simulink model "deneme"  (R2021a)
settings: Solver=FixedStepDiscrete  StartTime=0.0  StopTime=2  RelTol=1e-3  EnableMultiTasking=on
InitFcn:
  | pull_data ;
model workspace (MAT data in the model file):
  encoderResolution = 2000
  hallOffset = '0.5'
  indexOffset = 850
  polePairs = '4'
values from neighbouring files (symbols this model uses):
  bldc = mcb_bldc_param    [pull_data.m]
  dataType = 'single'    [pull_data.m]
  inverter = mcb_updateInverterParameters(bldc,inverter,target)    [pull_data.m]
  PI_params = mcb.internal.SetControllerParameters(bldc,inverter,PU_System,T_pwm,2*Ts,Ts_speed)    [pull_data.m]
  PU_System = mcb_SetPUSystem(bldc,inverter)    [pull_data.m]
  PWM_frequency = 20e3    (= 20000)    [pull_data.m]
  target = mcb_SetProcessorDetails('F28379D',PWM_frequency)    [pull_data.m]
  Ts = T_pwm    (= 5e-05)    [pull_data.m]
  Ts_motor = T_pwm/2    (= 2.5e-05)    [pull_data.m]
  Ts_motor_simscape = T_pwm/100    (= 5e-07)    [pull_data.m]
  Ts_simulink = T_pwm/2    (= 2.5e-05)    [pull_data.m]
  Ts_speed = 10*Ts    (= 0.0005)    [pull_data.m]
undefined symbols (not defined in the file or in its folder): Down, GPTRIP1SEL, GPTRIP2SEL, TZ1, TZ2, Up
libraries: nesl_utility x15, simulink x14, fl_lib x10, c2802xlib x9, mcbcontrolslib x8, c280xlib x6, mcbpositiondecoderlib x5, c2837xDlib x5, ee_lib x5, c2000lib x1, svdutilitieslib x1
(part 2 of 3)

== system deneme/Current Control/SCI (Code Generation)/Data_Logging ==
  note: Fast Serial Data Monitoring (32-bit)
  Data_Log : Inport
  Counter Limited : simulink/Sources/Counter Limited  uplimit=600-1  tsamp=-1
  Data : Subsystem  TreatAsAtomicUnit=on
  End : Subsystem  TreatAsAtomicUnit=on
  If : If  IfExpression=u1 == 0  ElseIfExpressions=u1 == 599
  Merge : Merge  Inputs=3
  Merge1 : Merge  Inputs=3
  Mux : Mux  Inputs=2
  Start : Subsystem  TreatAsAtomicUnit=on
  Width : Width  OutDataTypeMode=All ports same datatype  DataType=uint16
  SCI_Tx : Outport
  wires:
  If/3 -> Data/Action
  Data/1(Data_out) -> Merge/3
  Width/1 -> Data/2(Data_width), Start/2(Data_width), End/2(Data_width)
  Merge/1 -> Mux/1  "SCI_Tx_Data"
  Counter Limited/1 -> If/1
  Start/2(Iteration) -> Merge1/1
  Start/1(Data_out) -> Merge/1
  If/2 -> End/Action
  Merge1/1 -> Mux/2  "SCI_Tx_Iteration"
  If/1 -> Start/Action
  End/1(Data_out) -> Merge/2
  End/2(Iteration) -> Merge1/2
  Data/2(Iteration) -> Merge1/3
  Mux/1 -> SCI_Tx/1
  Data_Log/1 -> Width/1, Start/1(Data), End/1(Data), Data/1(Data)

== system deneme/Current Control/SCI (Code Generation)/While Iterator Subsystem ==
  Data : Inport
  Iteration : Inport  Port=2
  Add : Sum  Inputs=+-  OutDataTypeStr=Inherit: Same as first input
  Index Vector : MultiPortSwitch  Inputs=1
  SCI Transmit : c280xlib/SCI Transmit  sciModule=A  dataHead=''  dataTail=''  postInterrupt=off  numFifo=1
  While Iterator : WhileIterator  MaxIters=-1  WhileBlockType=do-while  ShowIterationPort=on  OutputDataType=int16
  wires:
  While Iterator/1 -> Add/2, Index Vector/1
  Data/1 -> Index Vector/2
  Index Vector/1 -> SCI Transmit/1
  Add/1 -> While Iterator/1
  Iteration/1 -> Add/1

== system deneme/Current Control/Sensor Driver Blocks/Sensor Driver Blocks (codegen) ==
  fb_sim : Inport
  Current Measurment : Subsystem
  Mux1 : Mux  Inputs=3
  Mux2 : Mux  Inputs=3
  Mux3 : Mux  Inputs=2
  Read Halls : Subsystem
  Terminator : Terminator
  eQEP : c280xlib/eQEP  useModule=eQEP1  pcInputmode=Quadrature-count  externalClockrate=2x resolution: Count the rising/falling edge  swapPolarityselection=Clockwise  qdfOutputport=off  qapPolarityselection=on  qbpPolarityselection=on  qipPolarityselection=on  qspPolarityselection=off  igatePolarityselection=off  sampleTime=-1  pcOutputport=on  pcMaximumvalue=2^16-1  indexInitializationcheck=off  indexInitializationevent=Rising edge  strobeInitializationcheck=off  strobeInitializationevent=Rising edge  softwareInitializationcheck=off  softwareInitializationsource=Set to init value at start up  softwareInitializationmode=on  pcInitialvalue=2147483648  pcResetmode=Reset on the first index event  ieloutputport=on  indexEventlatch=Falling edge  seloutputport=off  strobeEventlatch=Rising edge  pcefOutputport=off  enableEqepcapture=off  qctmrOutputport=off  qcprdOutputport=off  captureTimerprescaler=128  upEventprescaler=128  overflowErrorflag=off  directionErrorflag=off  captureTimerposition=On position counter read  unitTimerperiod=100000000  captureTimerlatch=off  capturePeriodlatch=off  positionCounterlatch=off  soenPolarityselection=off  spselPolarityselection=Index pin is used for sync output  compareValuesource=Specify via dialog  shadowMode=Load on QPOSCNT=0  compareValue=4294967295  syncOutputwidth=1  polaritySyncoutput=Active high  watchdogEnable=off  watchdogTimer=65535  outport1Datatype=auto  outport2Datatype=auto  outport3Datatype=auto  outport4Datatype=auto  outport5Datatype=auto  outport6Datatype=auto  outport7Datatype=auto  outport8Datatype=auto  outport9Datatype=auto  outport10Datatype=auto  outport11Datatype=auto  outport12Datatype=auto  eqepinterrupt_pce=off  eqepinterrupt_qpe=off  eqepinterrupt_qdc=off  eqepinterrupt_wto=off  eqepinterrupt_pcu=off  eqepinterrupt_pco=off  eqepinterrupt_pcr=off  eqepinterrupt_pcm=off  eqepinterrupt_sel=off  eqepinterrupt_iel=off  eqepinterrupt_uto=off  pheOutputport=off  watchdogOutputport=off  outport13Datatype=auto  outport14Datatype=auto
      settings: SourceProductBaseCode=TIC2000
  Iabc_Meas_ADC : Outport
  Hall_Meas : Outport  Port=2
  Qep_Meas : Outport  Port=3
  wires:
  Mux1/1 -> Iabc_Meas_ADC/1
  Current Measurment/1(IA) -> Mux1/1
  Current Measurment/2(IB) -> Mux1/2
  Current Measurment/3(IC) -> Mux1/3
  Read Halls/1(Hall_C) -> Mux2/1
  Read Halls/2(Hall_B) -> Mux2/2
  Read Halls/3(Hall_A) -> Mux2/3
  Mux2/1 -> Hall_Meas/1
  eQEP/1 -> Mux3/1
  eQEP/2 -> Mux3/2
  Mux3/1 -> Qep_Meas/1
  fb_sim/1 -> Terminator/1

== system deneme/Current Control/Sensor Driver Blocks/Sensor Driver Blocks (sim) ==
  fb_sim : Inport
  Bus Selector : BusSelector  OutputSignals=Iac_fb,Hall_fb,Pos_fb
  Iabc_Meas_ADC : Outport
  Hall_Meas : Outport  Port=2
  Qep_Meas : Outport  Port=3
  wires:
  Bus Selector/1 -> Iabc_Meas_ADC/1  "<Iac_fb>"
  Bus Selector/2 -> Hall_Meas/1  "<Hall_fb>"
  Bus Selector/3 -> Qep_Meas/1  "<Pos_fb>"
  fb_sim/1 -> Bus Selector/1

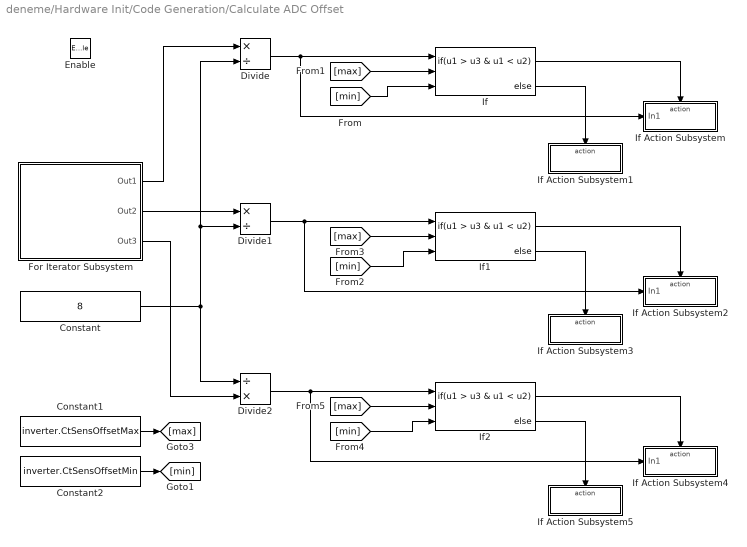
== system deneme/Hardware Init/Code Generation/Calculate ADC Offset  ==
  Enable : EnablePort
  Constant : Constant  Value=8
  Constant1 : Constant  Value=inverter.CtSensOffsetMax  OutDataTypeStr=Inherit: Inherit via back propagation
  Constant2 : Constant  Value=inverter.CtSensOffsetMin  OutDataTypeStr=Inherit: Inherit via back propagation
  Divide : Product  Inputs=*/  OutDataTypeStr=uint16
  Divide1 : Product  Inputs=*/  OutDataTypeStr=uint16
  Divide2 : Product  Inputs=/*  OutDataTypeStr=uint16
  For Iterator Subsystem : Subsystem  TreatAsAtomicUnit=on
  If : If  NumInputs=3  IfExpression=u1 > u3 & u1 < u2
  If Action Subsystem : Subsystem  TreatAsAtomicUnit=on
  If Action Subsystem1 : Subsystem  TreatAsAtomicUnit=on
  If Action Subsystem2 : Subsystem  TreatAsAtomicUnit=on
  If Action Subsystem3 : Subsystem  TreatAsAtomicUnit=on
  If Action Subsystem4 : Subsystem  TreatAsAtomicUnit=on
  If Action Subsystem5 : Subsystem  TreatAsAtomicUnit=on
  If1 : If  NumInputs=3  IfExpression=u1 > u3 & u1 < u2
  If2 : If  NumInputs=3  IfExpression=u1 > u3 & u1 < u2
  wires:
  Constant1/1 -> [max]
  [max] -> If1/2
  [min] -> If/3
  Divide1/1 -> If1/1, If Action Subsystem2/1(In1)
  [max] -> If/2
  [max] -> If2/2
  [min] -> If1/3
  Constant2/1 -> [min]
  [min] -> If2/3
  For Iterator Subsystem/1(Out1) -> Divide/1
  If2/1 -> If Action Subsystem4/Action
  If2/2 -> If Action Subsystem5/Action
  If1/2 -> If Action Subsystem3/Action
  If1/1 -> If Action Subsystem2/Action
  If/2 -> If Action Subsystem1/Action
  If/1 -> If Action Subsystem/Action
  For Iterator Subsystem/2(Out2) -> Divide1/1
  Divide2/1 -> If2/1, If Action Subsystem4/1(In1)
  Constant/1 -> Divide/2, Divide1/2, Divide2/1
  Divide/1 -> If Action Subsystem/1(In1), If/1
  For Iterator Subsystem/3(Out3) -> Divide2/2

== system deneme/Hardware Init/Code Generation/DRV Enable ==
  In : Inport
  Constant : Constant  OutDataTypeStr=Inherit: Inherit via back propagation
  DRV830x Enable : c2837xDlib/Digital Output  GPIO_Number=GPIO120~GPIO127  GPIO_Bit0=off  GPIO_BIT0_Toggle=off  GPIO_Bit1=off  GPIO_BIT1_Toggle=off  GPIO_Bit2=off  GPIO_BIT2_Toggle=off  GPIO_Bit3=off  GPIO_BIT3_Toggle=off  GPIO_Bit4=on  GPIO_BIT4_Toggle=off  GPIO_Bit5=off  GPIO_BIT5_Toggle=off  GPIO_Bit6=off  GPIO_BIT6_Toggle=off  GPIO_Bit7=off  GPIO_BIT7_Toggle=off
      settings: SourceProductBaseCode=TIC2000
  Demux : Demux  Outputs=2
  Display : Display
      settings: Format=hex (Stored Integer)
  Display1 : Display
      settings: Format=hex (Stored Integer)
  SPI Master Transfer2 : c280xlib/SPI Master Transfer  SPISelect=SPI_A  ClockPolarity=Rising_edge  ClockPhase=No_delay  SPIModule=uint32(0)  Mode=Master  BusSpeed=uint32(1000000)  FirstBitToTransfer=Most significant bit (MSB)  ClockMode=0  BlockFunction=Transfer  EnableRegisterAddress=off  RegisterAddress=0  OutputDataType=int8  OutputDataLength=1  DataBits=16  UseCustomSSPin=Provided by the SPI peripheral  ActiveLowSSPin=Active low  Pin=61
      settings: SourceProductBaseCode=TIC2000
  SPI Master Transfer3 : c280xlib/SPI Master Transfer  SPISelect=SPI_A  ClockPolarity=Rising_edge  ClockPhase=No_delay  SPIModule=uint32(0)  Mode=Master  BusSpeed=uint32(1000000)  FirstBitToTransfer=Most significant bit (MSB)  ClockMode=0  BlockFunction=Transfer  EnableRegisterAddress=off  RegisterAddress=0  OutputDataType=int8  OutputDataLength=1  DataBits=16  UseCustomSSPin=Provided by the SPI peripheral  ActiveLowSSPin=Active low  Pin=61
      settings: SourceProductBaseCode=TIC2000
  wires:
  Demux/2 -> SPI Master Transfer3/1
  SPI Master Transfer3/1 -> Display1/1
  SPI Master Transfer2/1 -> Display/1
  Demux/1 -> SPI Master Transfer2/1
  In/1 -> Demux/1
  Constant/1 -> DRV830x Enable/1

== system deneme/Hardware Init/Code Generation/Default ADC Offset ==
  Enable : EnablePort
  Constant : Constant  Value=inverter.CtSensAOffset  OutDataTypeStr=Inherit: Inherit via back propagation
  Constant1 : Constant  Value=inverter.CtSensBOffset  OutDataTypeStr=Inherit: Inherit via back propagation
  Constant2 : Constant  Value=inverter.CtSensCOffset  OutDataTypeStr=Inherit: Inherit via back propagation
  Data Store Write1 : DataStoreWrite  DataStoreName=IaOffset  IndexOptions=Index vector (dialog)  Indices=1  OutputSizes=1
  Data Store Write2 : DataStoreWrite  DataStoreName=IbOffset  IndexOptions=Index vector (dialog)  Indices=1  OutputSizes=1
  Data Store Write3 : DataStoreWrite  DataStoreName=IcOffset  IndexOptions=Index vector (dialog)  Indices=1  OutputSizes=1
  wires:
  Constant/1 -> Data Store Write1/1
  Constant1/1 -> Data Store Write2/1
  Constant2/1 -> Data Store Write3/1

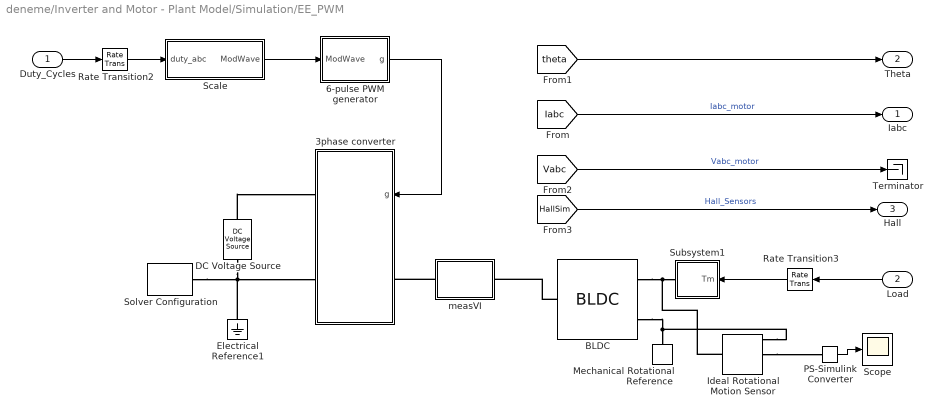
== system deneme/Inverter and Motor - Plant Model/Simulation/EE_PWM ==
  Duty_Cycles : Inport
  Load : Inport  Port=2
  3phase converter : Subsystem
  6-pulse PWM generator : Subsystem  mask{fs=PWM_frequency}
      mask prompts: fs "Carrier Frequency (Hz)"
  BLDC : ee_lib/Electromechanical/Permanent Magnet/BLDC  winding_type=ee.enum.statorconnection.wye  rotor_param=1  pm_flux_linkage=bldc.FluxPM Wb  theta_constant=pi /(2*bldc.p) rad  emf_max=9.6 V  DphiDtheta_tab=[0, -.1528, -.1528, .1528, .1528, 0] Wb/rad  back_emf_tab=[0, -9.6, -9.6, 9.6, 9.6, 0] V  rotor_angle_tab=[0, 7.5, 22.5, 37.5, 52.5, 60] deg  w_meas=600 rpm  nPolePairs=bldc.p  stator_param=ee.enum.statorparam.LdLqL0  machine_param=ee.enum.dqparameterization.constant  Ld=bldc.Ld H  Lq=bldc.Lq H  idVec=[-200, 0, 200] A  iqVec=[-200, 0, 200] A  LdMatrix=0.00022 * ones(3, 3) H  LqMatrix=0.00022 * ones(3, 3) H  L0=0.00016 H  Ls=0.0002 H  Lm=0 H  Ms=0.00002 H  Rs=bldc.Rs Ohm  zero_sequence=ee.enum.park.zerosequence.exclude  J=bldc.J kg*m^2  lam=bldc.B N*m/(rad/s)  axes_param=2  i_d_specify=off  i_d_priority=None  i_d=0 A  i_d_nominal_specify=off  i_d_nominal_unit=A  i_d_nominal_value=1  i_q_specify=off  i_q_priority=None  i_q=0 A  i_q_nominal_specify=off  i_q_nominal_unit=A  i_q_nominal_value=1  torque_specify=off  torque_priority=None  torque=0 N*m  torque_nominal_specify=off  torque_nominal_unit=N*m  torque_nominal_value=1  angular_velocity_specify=off  angular_velocity_priority=High  angular_velocity=0 rpm  angular_velocity_nominal_specify=off  angular_velocity_nominal_unit=rpm  angular_velocity_nominal_value=1  angular_position_specify=off  angular_position_priority=High  angular_position=0 deg  angular_position_nominal_specify=off  angular_position_nominal_unit=deg  angular_position_nominal_value=1  loss_param=ee.enum.ironloss.none  losses_oc=[0, 0, 0] W  losses_sc=[0, 0, 0] W  f_losses=60 Hz  Isc_losses=95 A  Tmeas=298.15 K  alpha=3.93e-3 1/K  alpha_flux=-0.001 1/K  stator_thermal_mass=100 J/K  rotor_thermal_mass=200 J/K  Rm_percent_rotor=90  Rd_percent_rotor=30  temperatureA_specify=off  temperatureA_priority=High  temperatureA=25 degC  temperatureA_nominal_specify=off  temperatureA_nominal_unit=degC  temperatureA_nominal_value=1  temperatureB_specify=off  temperatureB_priority=High  temperatureB=25 degC  temperatureB_nominal_specify=off  temperatureB_nominal_unit=degC  temperatureB_nominal_value=1  temperatureC_specify=off  temperatureC_priority=High  temperatureC=25 degC  temperatureC_nominal_specify=off  temperatureC_nominal_unit=degC  temperatureC_nominal_value=1  temperatureR_specify=off  temperatureR_priority=High  temperatureR=25 degC  temperatureR_nominal_specify=off  temperatureR_nominal_unit=degC  temperatureR_nominal_value=1
      settings: SourceProductBaseCode=PS  InternalSimscapePortConfiguration="{\"Bottom\":[],\"Left\":[{\"id\":\"N\",\"label\":\"~\",\"type\":\"foundation.electrical.three_phase\"}],\"Right\":[{\"id\":\"R\",\"label\":\"R\",\"type\":\"foundation.mechanical.rotational.rotational\"},{\"id\":\"C\",\"label\":\"C\",\"type\":\"foundation.mechanical.rotational.rotational\"}],\"Top\":[]}"
  DC Voltage Source : fl_lib/Electrical/Electrical Sources/DC Voltage Source  v0=inverter.V_dc V
  Electrical Reference1 : fl_lib/Electrical/Electrical Elements/Electrical Reference
  Ideal Rotational Motion Sensor : fl_lib/Mechanical/Mechanical Sensors/Ideal Rotational Motion Sensor  wrap_angle=simscape.enum.onoff.off  offset=0 rad
  Mechanical Rotational Reference : fl_lib/Mechanical/Rotational Elements/Mechanical Rotational Reference
  PS-Simulink Converter : nesl_utility/PS-Simulink Converter  PhysicalDomain=network_engine_domain  SubClassName=ps_output  LeftPortType=input  RightPortType=output  PseudoPeriodic=off  Frequencies=[]  Unit=inherit  AffineConversion=off
      settings: SourceProductBaseCode=PW,SS
  Rate Transition2 : RateTransition  Deterministic=off  OutPortSampleTime=Ts_motor_simscape
  Rate Transition3 : RateTransition  Deterministic=off  OutPortSampleTime=Ts_motor_simscape
  Scale : Subsystem
  Scope : Scope
  Solver Configuration : nesl_utility/Solver Configuration  PhysicalDomain=network_engine_domain  SubClassName=solver  LeftPortType=input  RightPortType=generic  Tones=[]  Harmonics=[]  SimulateNoise=off  Profile=off  UseLocalSampling=off  EnableSwitchedLinearOptims=on  FrequencyDomain=off  UseCCode=off  RelTol=0.001  AbsTol=1e-06  MinStep=1e-09  ToWorkspace=off  RevertToSquareIcSolve=off  NumHomotopyIterations=100  PhasorMode=off  PhasorModeNumHarmonics=1  DoDC=off  ResidualTolerance=1e-09  UseLocalSolver=on  LocalSolverChoice=NE_PARTITIONING_ADVANCER  LocalSolverSampleTime=Ts_motor_simscape  DoFixedCost=on  MaxNonlinIter=4  MaxModeIter=2  ComputeImpulses=off  ImpulseIterations=1  LinearAlgebra=auto  EquationFormulation=NE_TIME_EF  DelaysMemoryBudget=1024  AutomaticFiltering=on  FilteringTimeConstant=0.001  PartitionStorageMethod=AS_NEEDED  PartitionMemoryBudget=1024  PartitionMethod=ROBUST
      settings: SourceProductBaseCode=PW,SS
  Subsystem1 : Subsystem
  Terminator : Terminator
  measVI : Subsystem
  Iabc : Outport
  Theta : Outport  Port=2
  Hall : Outport  Port=3
  wires:
  Load/1 -> Rate Transition3/1
  [Iabc] -> Iabc/1  "Iabc_motor"
  [theta] -> Theta/1
  6-pulse PWM generator/1(g) -> 3phase converter/1(g)
  Scale/1(ModWave) -> 6-pulse PWM generator/1(ModWave)
  Duty_Cycles/1 -> Rate Transition2/1
  Rate Transition2/1 -> Scale/1(duty_abc)
  Rate Transition3/1 -> Subsystem1/1(Tm)
  [Vabc] -> Terminator/1  "Vabc_motor"
  [HallSim] -> Hall/1  "Hall_Sensors"
  PS-Simulink Converter/1 -> Scope/1
  connections:
  Solver Configuration/RConn1 -- 3phase converter/RConn2 -- DC Voltage Source/RConn1 -- Electrical Reference1/LConn1
  BLDC/LConn1 -- measVI/RConn1
  measVI/LConn1 -- 3phase converter/LConn1
  BLDC/RConn2 -- Ideal Rotational Motion Sensor/RConn1 -- Mechanical Rotational Reference/LConn1
  BLDC/RConn1 -- Ideal Rotational Motion Sensor/LConn1 -- Subsystem1/RConn1
  DC Voltage Source/LConn1 -- 3phase converter/RConn1
  Ideal Rotational Motion Sensor/RConn2 -- PS-Simulink Converter/LConn1

== system deneme/Inverter and Motor - Plant Model/Simulation/Load_Profile (Torque) ==
  Data Type Conversion : DataTypeConversion  OutDataTypeStr=single
  IIR Filter : mcbcontrolslib/IIR Filter  VariantControl=Low Pass Filter  VariantSelect=Low-pass  Filter_constant=0.01  advancedSettings=off  Ts=50e-6  cutOff_freq=32.1525
      settings: SourceProductBaseCode=MT
  "Motor Load reverse " : Constant  Value=-0.5*bldc.T_rated  OutDataTypeStr=dataType  SampleTime=-1
  Reversal : Step  Time=1.2
  Switch : Switch  Criteria=u2 > Threshold
  T_load : Step  Time=0.8  Before=0.05*bldc.T_rated  After=0.5*bldc.T_rated  SampleTime=Ts_simulink
  Load_Trq : Outport  VectorParamsAs1DForOutWhenUnconnected=off
  wires:
  Data Type Conversion/1 -> IIR Filter/1
  IIR Filter/1 -> Load_Trq/1
  Switch/1 -> Data Type Conversion/1
  Reversal/1 -> Switch/2
  T_load/1 -> Switch/3
  "Motor Load reverse "/1 -> Switch/1

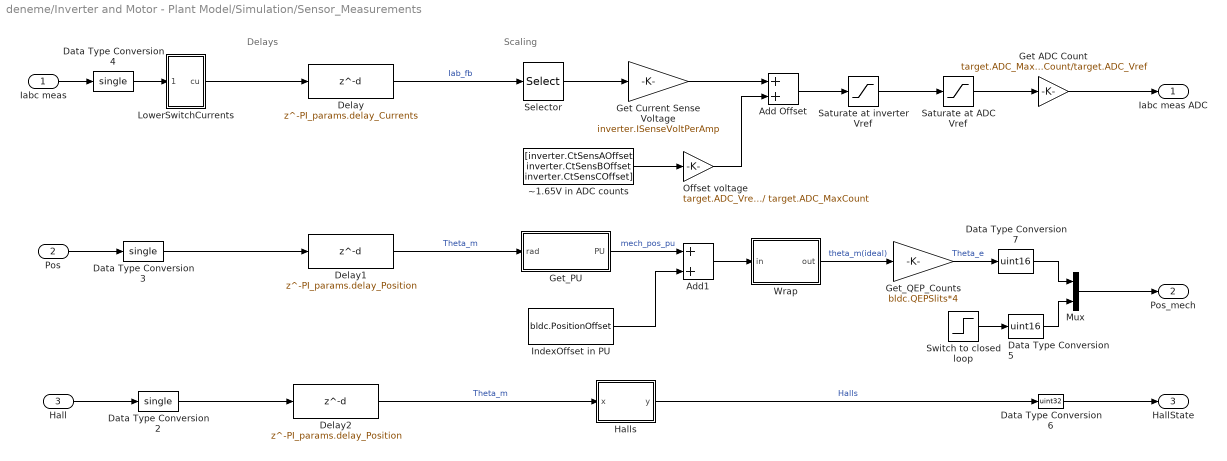
== system deneme/Inverter and Motor - Plant Model/Simulation/Sensor_Measurements ==
  note: Scaling
  note: Delays
  Iabc meas : Inport
  Pos : Inport  Port=2
  Hall : Inport  Port=3
  Add Offset : Sum  RndMeth=Simplest
  Add1 : Sum  RndMeth=Simplest
  Data Type Conversion2 : DataTypeConversion  OutDataTypeStr=single  RndMeth=Simplest
  Data Type Conversion3 : DataTypeConversion  OutDataTypeStr=single  RndMeth=Simplest
  Data Type Conversion4 : DataTypeConversion  OutDataTypeStr=single  RndMeth=Simplest
  Data Type Conversion5 : DataTypeConversion  OutDataTypeStr=uint16  RndMeth=Simplest
  Data Type Conversion6 : DataTypeConversion  OutDataTypeStr=uint32
  Data Type Conversion7 : DataTypeConversion  OutDataTypeStr=uint16  RndMeth=Simplest
  Delay : Delay  DelayLength=PI_params.delay_Currents
  Delay1 : Delay  DelayLength=PI_params.delay_Position
  Delay2 : Delay  DelayLength=PI_params.delay_Position
  Get ADC Count : Gain  Gain=target.ADC_MaxCount/target.ADC_Vref  OutMin=0  OutMax=target.ADC_MaxCount  OutDataTypeStr=uint16  RndMeth=Simplest
  Get Current Sense Voltage : Gain  Gain=inverter.ISenseVoltPerAmp  RndMeth=Simplest  OutDataTypeStr=Inherit: Same as input
  "Get_PU " : Subsystem
  Get_QEP_Counts : Gain  Gain=bldc.QEPSlits*4  OutDataTypeStr=uint16  RndMeth=Simplest
  Halls : Subsystem
  IndexOffset in PU : Constant  Value=bldc.PositionOffset  OutDataTypeStr=single  SampleTime=-1
  LowerSwitchCurrents : Subsystem
  Mux : Mux  Inputs=2
  Offset voltage : Gain  Gain=target.ADC_Vref / target.ADC_MaxCount  RndMeth=Simplest
  Saturate at ADC Vref : Saturate  UpperLimit=target.ADC_Vref  LowerLimit=0
  Saturate at inverter Vref : Saturate  UpperLimit=inverter.ISenseVref  LowerLimit=0
  Selector : Selector  InputPortWidth=3  IndexOptions=Index vector (dialog)  Indices=[1 2 3]  OutputSizes=1
  "Switch to closed loop " : Step  Time=0.1  SampleTime=Ts_motor
  Wrap : Subsystem
  ~1.65V in ADC counts : Constant  Value="[inverter.CtSensAOffset inverter.CtSensBOffset  inverter.CtSensCOffset]"  OutDataTypeStr=single  SampleTime=-1
  Iabc meas ADC : Outport  VectorParamsAs1DForOutWhenUnconnected=off
  Pos_mech : Outport  Port=2
  HallState : Outport  Port=3
  wires:
  Delay/1 -> Selector/1  "Iab_fb"
  Data Type Conversion4/1 -> LowerSwitchCurrents/1(In1)
  Iabc meas/1 -> Data Type Conversion4/1
  Data Type Conversion3/1 -> Delay1/1
  Pos/1 -> Data Type Conversion3/1
  Hall/1 -> Data Type Conversion2/1
  Data Type Conversion2/1 -> Delay2/1
  Delay2/1 -> Halls/1(x)  "Theta_m"
  Halls/1(y) -> Data Type Conversion6/1  "Halls"
  Data Type Conversion6/1 -> HallState/1
  LowerSwitchCurrents/1(cu) -> Delay/1
  Data Type Conversion5/1 -> Mux/2
  "Switch to closed loop "/1 -> Data Type Conversion5/1
  "Get_PU "/1(PU) -> Add1/1  "mech_pos_pu"
  IndexOffset in PU/1 -> Add1/2
  Mux/1 -> Pos_mech/1
  Data Type Conversion7/1 -> Mux/1
  Wrap/1(out) -> Get_QEP_Counts/1  "theta_m(ideal)"
  Get_QEP_Counts/1 -> Data Type Conversion7/1  "Theta_e"
  Add1/1 -> Wrap/1(in)
  Delay1/1 -> "Get_PU "/1(rad)  "Theta_m"
  Saturate at inverter Vref/1 -> Saturate at ADC Vref/1
  Add Offset/1 -> Saturate at inverter Vref/1
  ~1.65V in ADC counts/1 -> Offset voltage/1
  Offset voltage/1 -> Add Offset/2
  Get Current Sense Voltage/1 -> Add Offset/1
  Get ADC Count/1 -> Iabc meas ADC/1
  Saturate at ADC Vref/1 -> Get ADC Count/1
  Selector/1 -> Get Current Sense Voltage/1

== system deneme/Serial Receive/Code Generation/Data_Type_Fixed_Point ==
  SCI Receive : c280xlib/SCI Receive  sciModule=A  dataHead=''  dataTail=''  dataType=uint32  dataDim=2  initValue=0  errOption=Output the last received value  errValue=0  sampleTime=-1  outputStatus=off  postInterrupt=on  numFifo=4
      settings: SourceProductBaseCode=TIC2000
  Out1 : Outport
  wires:
  SCI Receive/1 -> Out1/1

== system deneme/Serial Receive/Code Generation/Data_Type_Float ==
  SCI Receive : c280xlib/SCI Receive  sciModule=A  dataHead=''  dataTail=''  dataType=single  dataDim=2  initValue=0  errOption=Output the last received value  errValue=0  sampleTime=-1  outputStatus=off  postInterrupt=on  numFifo=4
      settings: SourceProductBaseCode=TIC2000
  Out1 : Outport
  wires:
  SCI Receive/1 -> Out1/1

== system deneme/Serial Receive/Data_Conditioning_Rx/Data_Type_Fixed_Point ==
  In1 : Inport
  Data Type Conversion1 : DataTypeConversion  OutDataTypeStr=dataType  RndMeth=Simplest
  Data Type Conversion2 : DataTypeConversion  OutDataTypeStr=fixdt(1,32,28)  ConvertRealWorld=Stored Integer (SI)  RndMeth=Simplest
  Data Type Conversion3 : DataTypeConversion  OutDataTypeStr=uint16  RndMeth=Simplest
  Demux : Demux  Outputs=2
  Desired Speed : Outport
  Out2 : Outport  Port=2
  wires:
  In1/1 -> Demux/1
  Data Type Conversion1/1 -> Desired Speed/1
  Data Type Conversion2/1 -> Data Type Conversion1/1
  Demux/1 -> Data Type Conversion2/1
  Demux/2 -> Data Type Conversion3/1
  Data Type Conversion3/1 -> Out2/1

== system deneme/Serial Receive/Data_Conditioning_Rx/Data_Type_Float ==
  In1 : Inport
  Data Type Conversion2 : DataTypeConversion  OutDataTypeStr=uint16  RndMeth=Simplest
  Demux : Demux  Outputs=2
  Desired Speed : Outport
  Out2 : Outport  Port=2
  wires:
  In1/1 -> Demux/1
  Demux/1 -> Desired Speed/1
  Data Type Conversion2/1 -> Out2/1
  Demux/2 -> Data Type Conversion2/1

== system deneme/Serial Receive/Simulation/Data_Conditioning_Tx ==
  In1 : Inport
  In2 : Inport  Port=2
  Data_Type_Fixed_Point : Subsystem  VariantControl=~isequal(dataType, 'single')
  Data_Type_Float : Subsystem  VariantControl=isequal(dataType, 'single')
  Data : Outport

== system deneme/Serial Receive/Simulation/Parse ==
  Enable_PWM : Inport
  Debug_signals : Inport  Port=2
  Bitwise Operator : simulink/Logic and Bit Operations/Bitwise Operator  logicop=AND  UseBitMask=on  BitMask=hex2dec('0001')  BitMaskRealWorld=Stored Integer
  Bitwise Operator1 : simulink/Logic and Bit Operations/Bitwise Operator  logicop=AND  UseBitMask=on  BitMask=hex2dec('00F0')  BitMaskRealWorld=Stored Integer
  Shift Arithmetic1 : ArithShift  BitShiftNumber=-4
  Sum : Sum
  Data : Outport
  wires:
  Bitwise Operator/1 -> Sum/1
  Debug_signals/1 -> Shift Arithmetic1/1
  Sum/1 -> Data/1
  Shift Arithmetic1/1 -> Bitwise Operator1/1
  Enable_PWM/1 -> Bitwise Operator/1
  Bitwise Operator1/1 -> Sum/2

== system deneme/Current Control/Input Scaling/Convert ADC value to PU/Data_Type ==
  In1 : Inport
  Data_Type_Fixed_Point : Subsystem  VariantControl=~isequal(dataType,'single')
  Data_Type_Float : Subsystem  VariantControl=isequal(dataType,'single')
  Iab_meas_PU : Outport

== system deneme/Current Control/Input Scaling/Hall Feedback/Speed Counter ==
  Hall_State : Inport
  Constant4 : Constant  OutDataTypeStr=uint32  SampleTime=-1
  Delay : Delay  DelayLength=1  InitialCondition=1  ExternalReset=Level
      settings: InputPortMap=u0,r5
  Detect Change : simulink/Logic and Bit Operations/Detect Change  vinit=0  OutDataTypeStr=boolean
  Enabled Subsystem : Subsystem  TreatAsAtomicUnit=on
  Sum : Sum  Inputs=|++  AccumDataTypeStr=uint32  OutDataTypeStr=uint32  RndMeth=Simplest
  Unit Delay : UnitDelay  InitialCondition=1  SampleTime=-1  HasFrameUpgradeWarning=on
  Previous_Hall_State : Outport
  Speed_Count : Outport  Port=2
  wires:
  Delay/1 -> Unit Delay/1, Sum/2
  Constant4/1 -> Sum/1
  Sum/1 -> Delay/1
  Unit Delay/1 -> Enabled Subsystem/1(In1)
  Detect Change/1 -> Delay/2, Enabled Subsystem/Enable
  Enabled Subsystem/1(Speed_Count) -> Speed_Count/1
  Hall_State/1 -> Enabled Subsystem/2(Hall_State), Detect Change/1
  Enabled Subsystem/2(PrevHallState) -> Previous_Hall_State/1

== system deneme/Current Control/Input Scaling/Hall Feedback/Subsystem ==
  Hall_C : Inport
  Hall_B : Inport  Port=2
  Hall_A : Inport  Port=3
  Shift Arithmetic : ArithShift  BitShiftNumber=2  BitShiftDirection=Left
  Shift Arithmetic1 : ArithShift  BitShiftNumber=1  BitShiftDirection=Left
  Sum : Sum  Inputs=+++
  HallState : Outport
  wires:
  Shift Arithmetic/1 -> Sum/1
  Shift Arithmetic1/1 -> Sum/2
  Hall_C/1 -> Shift Arithmetic/1
  Hall_A/1 -> Sum/3
  Sum/1 -> HallState/1
  Hall_B/1 -> Shift Arithmetic1/1

== system deneme/Current Control/Input Scaling/QEP Feedback/ Calculate Position and Speed ==
  QEP_Position_Count : Inport
  QEP_Index_Latch : Inport  Port=2
  Offset : Inport  Port=3
  Delay : Delay  DelayLength=1
  IIR Filter : mcbcontrolslib/IIR Filter  VariantControl=Low Pass Filter  VariantSelect=Low-pass  Filter_constant=0.01  advancedSettings=off  Ts=50e-6  cutOff_freq=32.1525
      settings: SourceProductBaseCode=MT
  IndexFinder : Subsystem
  Mechanical to Electrical Position : mcbpositiondecoderlib/Mechanical to Electrical Position  NrPP=bldc.p  selectedRange=Per unit  MechOfstInputType=Input port  mechOffsetIn=0  maxAngleIn=1  InputDataType=dataType  VariantSelect=floating-point
      settings: SourceProductBaseCode=MT
  NOT : Logic  Operator=NOT  AllPortsSameDT=off  OutDataTypeStr=boolean
  Quadrature Decoder : mcbpositiondecoderlib/Quadrature Decoder  EncoderSlitsPerRevolution=bldc.QEPSlits  EncoderCountsPerSlit=4  CounterSize=16 bits  ExternalIndexCount=on  PositionUnit=Per unit  PositionDataType=dataType
      settings: SourceProductBaseCode=MT
  Speed Measurement : mcbpositiondecoderlib/Speed Measurement  PositionUnit=Per unit  SpeedCalculationMode=Time interval for speed calculation  SampleTimeAsync=Ts  MaximumApplicationSpeed=6000  SpeedResolution=5e-6  DelayLength=20  MaximumMeasurableSpeed=29999  MeasurableSpeedResolution=1.397e-05  SpeedUnit=Per unit based on dialog  PerUnitSpeed=PU_System.N_base  SpeedDataType=dataType
      settings: SourceProductBaseCode=MT
  Theta_e : Outport  VectorParamsAs1DForOutWhenUnconnected=off
  speed : Outport  Port=2  VectorParamsAs1DForOutWhenUnconnected=off
  IndexFound : Outport  Port=3  InitialOutput=0  VectorParamsAs1DForOutWhenUnconnected=off
  wires:
  Speed Measurement/1 -> IIR Filter/1
  Mechanical to Electrical Position/1 -> Theta_e/1
  QEP_Position_Count/1 -> Quadrature Decoder/1
  Quadrature Decoder/1 -> Speed Measurement/1, Mechanical to Electrical Position/1
  Offset/1 -> Mechanical to Electrical Position/2
  IIR Filter/1 -> speed/1
  Delay/1 -> NOT/1
  NOT/1 -> IndexFinder/Enable
  QEP_Index_Latch/1 -> IndexFinder/1(In1), Quadrature Decoder/2
  IndexFinder/1(Out1) -> Delay/1, IndexFound/1

== system deneme/Current Control/SCI (Code Generation)/Data_Conditioning_Tx/Data_Type_Fixed_Point ==
  In1 : Inport
  Data Type Conversion : DataTypeConversion  OutDataTypeStr=fixdt(1,32,28)  RndMeth=Simplest
  Data Type Conversion3 : DataTypeConversion  OutDataTypeStr=uint32  ConvertRealWorld=Stored Integer (SI)  RndMeth=Simplest
  Data_Log : Outport
  wires:
  In1/1 -> Data Type Conversion/1
  Data Type Conversion3/1 -> Data_Log/1
  Data Type Conversion/1 -> Data Type Conversion3/1

== system deneme/Current Control/SCI (Code Generation)/Data_Conditioning_Tx/Data_Type_Float ==
  In1 : Inport
  Byte Pack : svdutilitieslib/Byte Pack  maskPackedDataType=uint32  datatypes={'single'}  byteAlign=4  blockPlatform=tic2000
      settings: SourceProductBaseCode=ANDROID,ARDUINO,ML_ARDUINO,ECCORTEXA,ECCORTEXR,SC_BEAGLEBONE_BLUE,EC_FREEDOM_BOARD,EC_FRDM_K64F,INTEL_BLOCKSET,JETSONCPU,MICROBIT,NUCLEO,NVIDIA,PX4AUTOPILOTS,RASPPIIO,STMICRODIS,TIC2000,XILINX_BLOCKSET
  Data_Log : Outport
  wires:
  Byte Pack/1 -> Data_Log/1
  In1/1 -> Byte Pack/1

== system deneme/Current Control/SCI (Code Generation)/Data_Logging/Data ==
  Data : Inport
  Data_width : Inport  Port=2
  Action Port : ActionPort  ActionPortLabel=else
  Dummy : Constant  Value=hex2dec('0000')  OutDataTypeStr=uint32
  Mux : Mux  Inputs=2
  Data_out : Outport  VectorParamsAs1DForOutWhenUnconnected=off
  Iteration : Outport  Port=2  VectorParamsAs1DForOutWhenUnconnected=off
  wires:
  Data_width/1 -> Iteration/1
  Data/1 -> Mux/1
  Dummy/1 -> Mux/2
  Mux/1 -> Data_out/1

== system deneme/Current Control/SCI (Code Generation)/Data_Logging/End ==
  Data : Inport
  Data_width : Inport  Port=2
  Action Port : ActionPort  ActionPortLabel=elseif(u1 == 599)
  Bias : Bias  Bias=1
  End : Constant  Value=hex2dec('45454545')  OutDataTypeStr=uint32
  Mux : Mux  Inputs=2
  Data_out : Outport  VectorParamsAs1DForOutWhenUnconnected=off
  Iteration : Outport  Port=2  VectorParamsAs1DForOutWhenUnconnected=off
  wires:
  Data/1 -> Mux/1
  Data_width/1 -> Bias/1
  Bias/1 -> Iteration/1
  End/1 -> Mux/2
  Mux/1 -> Data_out/1

== system deneme/Current Control/SCI (Code Generation)/Data_Logging/Start ==
  Data : Inport
  Data_width : Inport  Port=2
  Action Port : ActionPort  ActionPortLabel=if(u1 == 0)
  Bias : Bias  Bias=1
  Mux : Mux  Inputs=2
  Start : Constant  Value=hex2dec('53535353')  OutDataTypeStr=uint32
  Data_out : Outport  VectorParamsAs1DForOutWhenUnconnected=off
  Iteration : Outport  Port=2  VectorParamsAs1DForOutWhenUnconnected=off
  wires:
  Data/1 -> Mux/2
  Data_width/1 -> Bias/1
  Bias/1 -> Iteration/1
  Start/1 -> Mux/1
  Mux/1 -> Data_out/1

== system deneme/Current Control/Sensor Driver Blocks/Sensor Driver Blocks (codegen)/Current Measurment ==
  ADC_A_IN2 : c2802xlib/ADC  blkParamProc=C2000_Type4  ADCModule=A  samplingMode=Single sample mode  ADCResolution=12-bit (Single-ended input)  useSOC1=SOC0  useSOC2=SOC0_SOC1  SOCAcquisitionWindow=15  SOCTriggerSource=ePWM1_ADCSOCA  SOCInterruptTrigger=No ADCINT  Ts=-1  dType=uint16  postInterrupt=on  interruptSel=ADCINT1  ADCINTContinuous=on  endma=off  chdma=1  conv1=ADCINA0  conv2=ADCINA0 and ADCINB0  conv1_Type4=ADCIN2  conv2_Type4=ADCIN0 and ADCIN1
  ADC_B_IN2 : c2802xlib/ADC  blkParamProc=C2000_Type4  ADCModule=B  samplingMode=Single sample mode  ADCResolution=12-bit (Single-ended input)  useSOC1=SOC0  useSOC2=SOC0_SOC1  SOCAcquisitionWindow=15  SOCTriggerSource=ePWM1_ADCSOCA  SOCInterruptTrigger=No ADCINT  Ts=-1  dType=uint16  postInterrupt=off  interruptSel=ADCINT1  ADCINTContinuous=on  endma=off  chdma=1  conv1=ADCINA0  conv2=ADCINA0 and ADCINB0  conv1_Type4=ADCIN2  conv2_Type4=ADCIN0 and ADCIN1
  ADC_C_IN2 : c2802xlib/ADC  blkParamProc=C2000_Type4  ADCModule=C  samplingMode=Single sample mode  ADCResolution=12-bit (Single-ended input)  useSOC1=SOC0  useSOC2=SOC0_SOC1  SOCAcquisitionWindow=15  SOCTriggerSource=ePWM1_ADCSOCA  SOCInterruptTrigger=No ADCINT  Ts=-1  dType=uint16  postInterrupt=off  interruptSel=ADCINT1  ADCINTContinuous=on  endma=off  chdma=1  conv1=ADCINA0  conv2=ADCINA0 and ADCINB0  conv1_Type4=ADCIN2  conv2_Type4=ADCIN0 and ADCIN1
  IA : Outport
  IB : Outport  Port=2
  IC : Outport  Port=3
  wires:
  ADC_A_IN2/1 -> IC/1
  ADC_C_IN2/1 -> IA/1
  ADC_B_IN2/1 -> IB/1

== system deneme/Current Control/Sensor Driver Blocks/Sensor Driver Blocks (codegen)/Read Halls ==
  Demux : Demux  Outputs=2
  Digital Input : c2837xDlib/Digital Input  GPIO_Number=GPIO48~GPIO55  GPIO_Bit0=off  GPIO_Bit1=off  GPIO_Bit2=off  GPIO_Bit3=off  GPIO_Bit4=off  GPIO_Bit5=off  GPIO_Bit6=on  GPIO_Bit7=on  sampleTime=-1  dataType=uint32  GPIO_Bit0_Qualification=Sync to SYSCLKOUT  GPIO_Bit1_Qualification=Sync to SYSCLKOUT  GPIO_Bit2_Qualification=Sync to SYSCLKOUT  GPIO_Bit3_Qualification=Sync to SYSCLKOUT  GPIO_Bit4_Qualification=Sync to SYSCLKOUT  GPIO_Bit5_Qualification=Sync to SYSCLKOUT  GPIO_Bit6_Qualification=Sync to SYSCLKOUT  GPIO_Bit7_Qualification=Sync to SYSCLKOUT  Qualification_Period=-1
      settings: SourceProductBaseCode=TIC2000
  Digital Input1 : c2837xDlib/Digital Input  GPIO_Number=GPIO56~GPIO63  GPIO_Bit0=off  GPIO_Bit1=on  GPIO_Bit2=off  GPIO_Bit3=off  GPIO_Bit4=off  GPIO_Bit5=off  GPIO_Bit6=off  GPIO_Bit7=off  sampleTime=-1  dataType=uint32  GPIO_Bit0_Qualification=Sync to SYSCLKOUT  GPIO_Bit1_Qualification=Sync to SYSCLKOUT  GPIO_Bit2_Qualification=Sync to SYSCLKOUT  GPIO_Bit3_Qualification=Sync to SYSCLKOUT  GPIO_Bit4_Qualification=Sync to SYSCLKOUT  GPIO_Bit5_Qualification=Sync to SYSCLKOUT  GPIO_Bit6_Qualification=Sync to SYSCLKOUT  GPIO_Bit7_Qualification=Sync to SYSCLKOUT  Qualification_Period=-1
      settings: SourceProductBaseCode=TIC2000
  Hall_C : Outport
  Hall_B : Outport  Port=2
  Hall_A : Outport  Port=3
  wires:
  Digital Input/1 -> Demux/1
  Digital Input1/1 -> Hall_C/1
  Demux/2 -> Hall_B/1
  Demux/1 -> Hall_A/1

== system deneme/Hardware Init/Code Generation/Calculate ADC Offset /For Iterator Subsystem ==
  ADC_A_IN0 : c2802xlib/ADC  Priority=20  blkParamProc=C2000_Type4  ADCModule=C  samplingMode=Single sample mode  ADCResolution=12-bit (Single-ended input)  useSOC1=SOC2  useSOC2=SOC0_SOC1  SOCAcquisitionWindow=15  SOCTriggerSource=Software  SOCInterruptTrigger=No ADCINT  Ts=-1  dType=uint16  postInterrupt=off  interruptSel=ADCINT1  ADCINTContinuous=on  endma=off  chdma=1  conv1=ADCINA0  conv2=ADCINA0 and ADCINB0  conv1_Type4=ADCIN2  conv2_Type4=ADCIN0 and ADCIN1
  ADC_B_IN0 : c2802xlib/ADC  Priority=20  blkParamProc=C2000_Type4  ADCModule=B  samplingMode=Single sample mode  ADCResolution=12-bit (Single-ended input)  useSOC1=SOC2  useSOC2=SOC0_SOC1  SOCAcquisitionWindow=15  SOCTriggerSource=Software  SOCInterruptTrigger=No ADCINT  Ts=-1  dType=uint16  postInterrupt=off  interruptSel=ADCINT1  ADCINTContinuous=on  endma=off  chdma=1  conv1=ADCINA0  conv2=ADCINA0 and ADCINB0  conv1_Type4=ADCIN2  conv2_Type4=ADCIN0 and ADCIN1
  ADC_C_IN0 : c2802xlib/ADC  Priority=20  blkParamProc=C2000_Type4  ADCModule=A  samplingMode=Single sample mode  ADCResolution=12-bit (Single-ended input)  useSOC1=SOC2  useSOC2=SOC0_SOC1  SOCAcquisitionWindow=15  SOCTriggerSource=Software  SOCInterruptTrigger=No ADCINT  Ts=-1  dType=uint16  postInterrupt=off  interruptSel=ADCINT1  ADCINTContinuous=on  endma=off  chdma=1  conv1=ADCINA0  conv2=ADCINA0 and ADCINB0  conv1_Type4=ADCIN2  conv2_Type4=ADCIN0 and ADCIN1
  For Iterator : ForIterator  IterationLimit=16  IterationVariableDataType=uint16
  If : If  IfExpression=u1 > 8  ShowElse=off
  If Action Subsystem : Subsystem  TreatAsAtomicUnit=on
  Out1 : Outport
  Out2 : Outport  Port=2
  Out3 : Outport  Port=3
  wires:
  For Iterator/1 -> If/1
  ADC_A_IN0/1 -> If Action Subsystem/1(In1)
  ADC_B_IN0/1 -> If Action Subsystem/2(In2)
  If Action Subsystem/1(Out1) -> Out1/1
  If Action Subsystem/2(Out2) -> Out2/1
  If/1 -> If Action Subsystem/Action
  ADC_C_IN0/1 -> If Action Subsystem/3(In3)
  If Action Subsystem/3(Out3) -> Out3/1

== system deneme/Hardware Init/Code Generation/Calculate ADC Offset /If Action Subsystem ==
  In1 : Inport
  Action Port : ActionPort  ActionPortLabel=if(u1 > 1500 & u1 < 2500)
  Data Store Write1 : DataStoreWrite  DataStoreName=IaOffset  IndexOptions=Index vector (dialog)  Indices=1  OutputSizes=1
  wires:
  In1/1 -> Data Store Write1/1

== system deneme/Hardware Init/Code Generation/Calculate ADC Offset /If Action Subsystem1 ==
  Action Port : ActionPort  ActionPortLabel=else
  Constant : Constant  Value=inverter.CtSensAOffset  OutDataTypeStr=Inherit: Inherit via back propagation
  Data Store Write1 : DataStoreWrite  DataStoreName=IaOffset  IndexOptions=Index vector (dialog)  Indices=1  OutputSizes=1
  wires:
  Constant/1 -> Data Store Write1/1

== system deneme/Hardware Init/Code Generation/Calculate ADC Offset /If Action Subsystem2 ==
  In1 : Inport
  Action Port : ActionPort  ActionPortLabel=if(u1 > 1500 & u1 < 2500)
  Data Store Write2 : DataStoreWrite  DataStoreName=IbOffset  IndexOptions=Index vector (dialog)  Indices=1  OutputSizes=1
  wires:
  In1/1 -> Data Store Write2/1

== system deneme/Hardware Init/Code Generation/Calculate ADC Offset /If Action Subsystem3 ==
  Action Port : ActionPort  ActionPortLabel=else
  Constant1 : Constant  Value=inverter.CtSensBOffset  OutDataTypeStr=Inherit: Inherit via back propagation
  Data Store Write2 : DataStoreWrite  DataStoreName=IbOffset  IndexOptions=Index vector (dialog)  Indices=1  OutputSizes=1
  wires:
  Constant1/1 -> Data Store Write2/1

== system deneme/Hardware Init/Code Generation/Calculate ADC Offset /If Action Subsystem4 ==
  In1 : Inport
  Action Port : ActionPort  ActionPortLabel=if(u1 > 1500 & u1 < 2500)
  Data Store Write2 : DataStoreWrite  DataStoreName=IcOffset  IndexOptions=Index vector (dialog)  Indices=1  OutputSizes=1
  wires:
  In1/1 -> Data Store Write2/1

== system deneme/Hardware Init/Code Generation/Calculate ADC Offset /If Action Subsystem5 ==
  Action Port : ActionPort  ActionPortLabel=else
  Constant1 : Constant  Value=inverter.CtSensCOffset  OutDataTypeStr=Inherit: Inherit via back propagation
  Data Store Write2 : DataStoreWrite  DataStoreName=IcOffset  IndexOptions=Index vector (dialog)  Indices=1  OutputSizes=1
  wires:
  Constant1/1 -> Data Store Write2/1

== system deneme/Inverter and Motor - Plant Model/Simulation/EE_PWM/3phase converter ==
  g : Inport
  Demux : Demux  Outputs=6
  Inverter : ee_lib/Semiconductors & Converters/Converters/Converter (Three-Phase)  device_type=ee.enum.converters.switchingdevice.mosfet  Vf=0.8 V  Ron=0.001 Ohm  Rds="inverter.Rds_on  Ohm"  Goff=1e-5 1/Ohm  Vth=0.7 V  Vgt=1 V  Vgt_off=-1 V  Ih=1 A  diode_param=ee.enum.converters.protectiondiode.nodynamics  diode_Vf=0.7 V  diode_Ron="inverter.Rds_on  Ohm"  diode_Goff=1e-5 1/Ohm  diode_C=50 nF  diode_iRM=-235 A  diode_iF=300 A  diode_idot=-50 A/us  diode_trr_param=ee.enum.converters.diodetrr.trr_factor  diode_trr_factor=3  diode_trr=15 us  diode_Qrr=1.5e+3 s*uA  snubber_type=ee.enum.converters.snubber.exclude  Rs=0.1 Ohm  Cs=1e-7 F
      settings: SourceProductBaseCode=PS
  Simulink-PS Converter{,1..5} (6 alike) : nesl_utility/Simulink-PS Converter  PhysicalDomain=network_engine_domain  SubClassName=ps_input  LeftPortType=input  RightPortType=output  PseudoPeriodic=off  Frequencies=[]  NoiseDistribution=none  NoiseParameters=[]  Unit=1  AffineConversion=off  FilteringAndDerivatives=provide  SimscapeFilterOrder=1  InputFilterTimeConstant=0.001  UdotUserProvided=0
      settings: SourceProductBaseCode=PW,SS
  Six-Pulse Gate Multiplexer : ee_lib/Semiconductors & Converters/Converters/Six-Pulse Gate Multiplexer  R=0 Ohm
      settings: SourceProductBaseCode=PS  InternalSimscapePortConfiguration="{\"Bottom\":[],\"Left\":[{\"id\":\"GaH\",\"label\":\"Ga(H)\",\"type\":\"input\"},{\"id\":\"GaL\",\"label\":\"Ga(L)\",\"type\":\"input\"},{\"id\":\"GbH\",\"label\":\"Gb(H)\",\"type\":\"input\"},{\"id\":\"GbL\",\"label\":\"Gb(L)\",\"type\":\"input\"},{\"id\":\"GcH\",\"label\":\"Gc(H)\",\"type\":\"input\"},{\"id\":\"GcL\",\"label\":\"Gc(L)\",\"type\":\"input\"}],\"Right\":[{\"id\":\"p\",\"label\":\"G\",\"type\":\"foundation.electrical.twelve_phase\"}],\"Top\":[]}"
  + : PMIOPort  Side=Right
  ~ : PMIOPort  Port=2  Side=Left
  - : PMIOPort  Port=3  Side=Right
  wires:
  g/1 -> Demux/1
  Demux/1 -> Simulink-PS Converter/1
  Demux/2 -> Simulink-PS Converter1/1
  Demux/3 -> Simulink-PS Converter2/1
  Demux/4 -> Simulink-PS Converter3/1
  Demux/6 -> Simulink-PS Converter5/1
  Demux/5 -> Simulink-PS Converter4/1
  connections:
  Simulink-PS Converter/RConn1 -- Six-Pulse Gate Multiplexer/LConn1
  Inverter/RConn2 -- -/RConn1
  Inverter/RConn1 -- +/RConn1
  Inverter/LConn2 -- ~/RConn1
  Inverter/LConn1 -- Six-Pulse Gate Multiplexer/RConn1
  Simulink-PS Converter1/RConn1 -- Six-Pulse Gate Multiplexer/LConn2
  Simulink-PS Converter2/RConn1 -- Six-Pulse Gate Multiplexer/LConn3
  Simulink-PS Converter3/RConn1 -- Six-Pulse Gate Multiplexer/LConn4
  Simulink-PS Converter4/RConn1 -- Six-Pulse Gate Multiplexer/LConn5
  Simulink-PS Converter5/RConn1 -- Six-Pulse Gate Multiplexer/LConn6

== system deneme/Inverter and Motor - Plant Model/Simulation/EE_PWM/6-pulse PWM generator ==
  ModWave : Inport
  Relay : Relay
  Repeating Sequence Interpolated : simulink/Sources/Repeating Sequence Interpolated  OutValues="[0 1   0].'"  TimeValues=0.25/fs*[0 2 4].'  LookUpMeth=Interpolation-Use End Values  tsamp=Ts_motor_simscape  OutMin=[]  OutMax=[]  OutDataTypeStr=double  OutputDataTypeScalingMode=double  OutDataType=fixdt(0,8)  OutScaling=2^-10
  Sum : Sum  Inputs=|+-
  g : Outport
  wires:
  Relay/1 -> g/1
  Repeating Sequence Interpolated/1 -> Sum/2  "carrier"
  Sum/1 -> Relay/1
  ModWave/1 -> Sum/1

== system deneme/Inverter and Motor - Plant Model/Simulation/EE_PWM/Scale ==
  duty_abc : Inport
  Constant : Constant  Value=0  OutDataTypeStr=single  SampleTime=Ts_motor_simscape
  Data Type Conversion : DataTypeConversion
  Gain : Gain
  Rate Transition : RateTransition
  Sum : Sum  Inputs=|++
  ModWave : Outport
  wires:
  Gain/1 -> Data Type Conversion/1
  Data Type Conversion/1 -> Rate Transition/1
  Rate Transition/1 -> ModWave/1  "ModWave"
  duty_abc/1 -> Sum/1  "beforeGain"
  Constant/1 -> Sum/2
  Sum/1 -> Gain/1

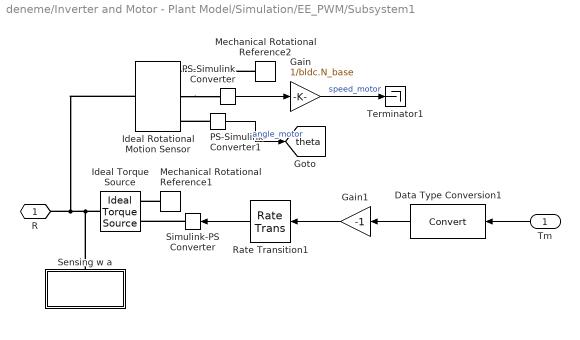
== system deneme/Inverter and Motor - Plant Model/Simulation/EE_PWM/Subsystem1 ==
  Tm : Inport
  Data Type Conversion1 : DataTypeConversion
  Gain : Gain  Gain=1/bldc.N_base
  Gain1 : Gain  Gain=-1
  Ideal Rotational Motion Sensor : fl_lib/Mechanical/Mechanical Sensors/Ideal Rotational Motion Sensor  wrap_angle=simscape.enum.onoff.off  offset=0 rad
  Ideal Torque Source : fl_lib/Mechanical/Mechanical Sources/Ideal Torque Source
  Mechanical Rotational Reference1 : fl_lib/Mechanical/Rotational Elements/Mechanical Rotational Reference
  Mechanical Rotational Reference2 : fl_lib/Mechanical/Rotational Elements/Mechanical Rotational Reference
  PS-Simulink Converter : nesl_utility/PS-Simulink Converter  PhysicalDomain=network_engine_domain  SubClassName=ps_output  LeftPortType=input  RightPortType=output  PseudoPeriodic=off  Frequencies=[]  Unit=rpm  AffineConversion=off
      settings: SourceProductBaseCode=PW,SS
  PS-Simulink Converter1 : nesl_utility/PS-Simulink Converter  PhysicalDomain=network_engine_domain  SubClassName=ps_output  LeftPortType=input  RightPortType=output  PseudoPeriodic=off  Frequencies=[]  Unit=inherit  AffineConversion=off
      settings: SourceProductBaseCode=PW,SS
  Rate Transition1 : RateTransition
  Sensing w a : Subsystem
      mask Display: disp('w,Hall')
  Simulink-PS Converter : nesl_utility/Simulink-PS Converter  PhysicalDomain=network_engine_domain  SubClassName=ps_input  LeftPortType=input  RightPortType=output  PseudoPeriodic=off  Frequencies=[]  NoiseDistribution=none  NoiseParameters=[]  Unit=N*m  AffineConversion=off  FilteringAndDerivatives=provide  SimscapeFilterOrder=1  InputFilterTimeConstant=0.001  UdotUserProvided=0
      settings: SourceProductBaseCode=PW,SS
  Terminator1 : Terminator
  "R " : PMIOPort  Side=Right
  tag scope: theta=global
  wires:
  Gain1/1 -> Rate Transition1/1
  Rate Transition1/1 -> Simulink-PS Converter/1
  Data Type Conversion1/1 -> Gain1/1
  Tm/1 -> Data Type Conversion1/1
  PS-Simulink Converter/1 -> Gain/1
  Gain/1 -> Terminator1/1  "speed_motor"
  PS-Simulink Converter1/1 -> [theta]  "angle_motor"
  connections:
  Mechanical Rotational Reference1/LConn1 -- Ideal Torque Source/RConn2
  Simulink-PS Converter/RConn1 -- Ideal Torque Source/RConn1
  Ideal Torque Source/LConn1 -- "R "/RConn1 -- Ideal Rotational Motion Sensor/LConn1 -- Sensing w a/LConn1
  Ideal Rotational Motion Sensor/RConn2 -- PS-Simulink Converter/LConn1
  PS-Simulink Converter1/LConn1 -- Ideal Rotational Motion Sensor/RConn3
  Mechanical Rotational Reference2/LConn1 -- Ideal Rotational Motion Sensor/RConn1

== system deneme/Inverter and Motor - Plant Model/Simulation/EE_PWM/measVI ==
  Current Sensor (Three-Phase) : ee_lib/Sensors & Transducers/Current Sensor (Three-Phase)
  Line Voltage Sensor (Three-Phase) : ee_lib/Sensors & Transducers/Line Voltage Sensor (Three-Phase)
      settings: SourceProductBaseCode=PS
  PS-Simulink Converter2 : nesl_utility/PS-Simulink Converter  PhysicalDomain=network_engine_domain  SubClassName=ps_output  LeftPortType=input  RightPortType=output  PseudoPeriodic=off  Frequencies=[]  Unit=inherit  AffineConversion=off
      settings: SourceProductBaseCode=PW,SS
  PS-Simulink Converter3 : nesl_utility/PS-Simulink Converter  PhysicalDomain=network_engine_domain  SubClassName=ps_output  LeftPortType=input  RightPortType=output  PseudoPeriodic=off  Frequencies=[]  Unit=inherit  AffineConversion=off
      settings: SourceProductBaseCode=PW,SS
  ~1 : PMIOPort  Side=Left
  ~2 : PMIOPort  Port=2  Side=Right
  tag scope: Iabc=global, Vabc=global
  wires:
  PS-Simulink Converter2/1 -> [Vabc]  "Vabc"
  PS-Simulink Converter3/1 -> [Iabc]  "Iabc"
  connections:
  Current Sensor (Three-Phase)/RConn1 -- PS-Simulink Converter3/LConn1
  PS-Simulink Converter2/LConn1 -- Line Voltage Sensor (Three-Phase)/RConn1
  Current Sensor (Three-Phase)/RConn2 -- ~2/RConn1
  Line Voltage Sensor (Three-Phase)/LConn1 -- ~1/RConn1 -- Current Sensor (Three-Phase)/LConn1

== system deneme/Inverter and Motor - Plant Model/Simulation/Sensor_Measurements/Get_PU  ==
  rad : Inport
  Constant2 : Constant  Value=2*pi  OutDataTypeStr=single  SampleTime=-1
  Get_PU : Gain  Gain=1/(2*pi)  RndMeth=Simplest  OutDataTypeStr=Inherit: Same as input
  Mod : Math  Operator=mod  SaturateOnIntegerOverflow=on
  PU : Outport  VectorParamsAs1DForOutWhenUnconnected=off
  wires:
  rad/1 -> Mod/1
  Constant2/1 -> Mod/2
  Mod/1 -> Get_PU/1
  Get_PU/1 -> PU/1  "mech_pos_pu"

== system deneme/Inverter and Motor - Plant Model/Simulation/Sensor_Measurements/Halls ==
  x : Inport
  Gain : Gain  Gain=[4 2 1]  Multiplication=Matrix(K*u)
  Hall Signals HW : Subsystem
  Hall State Plant to HW : Subsystem
  Sum of Elements : Sum  Inputs=+
  y : Outport  VectorParamsAs1DForOutWhenUnconnected=off
  wires:
  Gain/1 -> Sum of Elements/1
  x/1 -> Gain/1
  Sum of Elements/1 -> Hall State Plant to HW/1(HallStatePlant)
  Hall State Plant to HW/1(HallstateHw) -> Hall Signals HW/1(HallState)  "HallState"
  Hall Signals HW/1(Hall Signals) -> y/1

== system deneme/Inverter and Motor - Plant Model/Simulation/Sensor_Measurements/LowerSwitchCurrents ==
  In1 : Inport
  Constant : Constant  Value=0
  Switch : Switch  Criteria=u2 > Threshold
  cu : Outport
  wires:
  Constant/1 -> Switch/1
  In1/1 -> Switch/2, Switch/3
  Switch/1 -> cu/1  "cu"

== system deneme/Inverter and Motor - Plant Model/Simulation/Sensor_Measurements/Wrap ==
  in : Inport
  Constant2 : Constant  OutDataTypeStr=single  SampleTime=-1
  Mod : Math  Operator=mod  SaturateOnIntegerOverflow=on
  out : Outport  VectorParamsAs1DForOutWhenUnconnected=off
  wires:
  in/1 -> Mod/1
  Constant2/1 -> Mod/2
  Mod/1 -> out/1

== system deneme/Serial Receive/Simulation/Data_Conditioning_Tx/Data_Type_Fixed_Point ==
  In1 : Inport
  In2 : Inport  Port=2
  Data Type Conversion : DataTypeConversion  OutDataTypeStr=fixdt(1,32,28)  RndMeth=Simplest
  Data Type Conversion1 : DataTypeConversion  OutDataTypeStr=uint32  RndMeth=Simplest
  Data Type Conversion3 : DataTypeConversion  OutDataTypeStr=uint32  ConvertRealWorld=Stored Integer (SI)  RndMeth=Simplest
  Mux : Mux  Inputs=2
  Data : Outport
  wires:
  In1/1 -> Data Type Conversion/1
  Data Type Conversion3/1 -> Mux/1
  Data Type Conversion/1 -> Data Type Conversion3/1
  In2/1 -> Data Type Conversion1/1
  Data Type Conversion1/1 -> Mux/2
  Mux/1 -> Data/1

== system deneme/Serial Receive/Simulation/Data_Conditioning_Tx/Data_Type_Float ==
  In1 : Inport
  In2 : Inport  Port=2
  Data Type Conversion2 : DataTypeConversion  OutDataTypeStr=single  RndMeth=Simplest
  Mux : Mux  Inputs=2
  Data : Outport
  wires:
  In1/1 -> Mux/1
  Mux/1 -> Data/1
  In2/1 -> Data Type Conversion2/1
  Data Type Conversion2/1 -> Mux/2

== system deneme/Current Control/Input Scaling/Convert ADC value to PU/Data_Type/Data_Type_Fixed_Point ==
  In1 : Inport
  Data Type Conversion : DataTypeConversion  OutDataTypeStr=fixdt(1,32,17)  ConvertRealWorld=Stored Integer (SI)  RndMeth=Simplest
  Data Type Conversion1 : DataTypeConversion  OutDataTypeStr=dataType  RndMeth=Simplest
  Q17 per unit conversion : ArithShift  BitShiftNumber=-6
  Iab_meas_PU : Outport
  wires:
  In1/1 -> Q17 per unit conversion/1
  Data Type Conversion1/1 -> Iab_meas_PU/1
  Data Type Conversion/1 -> Data Type Conversion1/1
  Q17 per unit conversion/1 -> Data Type Conversion/1
